simulink model "Joystick"  (R2017a)
settings: Solver=ode2  StartTime=0.0  StopTime=inf  FixedStep=0.001  RelTol=1e-3  EnableMultiTasking=on
model workspace (MAT data in the model file):
  Sig = Simulink.Signal
  Sig.DataType = 'auto'
  Sig.Dimensions = -1
  Sig.DimensionsMode = 'auto'
  Sig.Complexity = 'auto'
  Sig.SampleTime = -1
  Sig.SamplingMode = 'auto'
  video_step_size = 0.06
libraries: quarc_library x1
settings Model: SimulationMode=external  Creator=Admin  LastModifiedBy=mbohra
settings SolverCC: PositivePriorityOrder=on
settings OptimizationCC: LifeSpan=inf
settings DebuggingCC: ParameterPrecisionLossMsg=none  SFUnexpectedBacktrackingDiag=warning  SFNoUnconditionalDefaultTransitionDiag=warning  SFExecutionAtInitializationDiag=none
settings HardwareCC: ProdBitPerLong=64  ProdLargestAtomicFloat=None  ProdHWDeviceType=Intel->x86-64
settings RTWCC: SystemTargetFile=quarc_linux_x64.tlc  TemplateMakefile=quarc_linux_x64_tmf  Description=QUARC Linux x64 Target
settings STFCustomTargetCC: TargetLibSuffix=.a  TargetPreCompLibLocation=C:\PROGRA~3\QUARC\lib\2017a\LINUX_~1\release  ConcurrentExecutionCompliant=on  SystemTargetFile=quarc_linux_x64.tlc
settings GRTTargetCC: TargetLibSuffix=.a  TargetPreCompLibLocation=C:\PROGRA~3\QUARC\lib\2017a\LINUX_~1\release  TargetLangStandard=C89/C90 (ANSI)  ParMdlRefBuildCompliant=off  CompOptLevelCompliant=off  CombineOutputUpdateFcns=off  MatFileLogging=off  CPPClassGenCompliant=off  GRTInterface=on  UseToolchainInfoCompliant=off  ExtMode=on  ExtModeMexFile=quarc_comm  ExtModeMexArgs='-w -d /tmp -uri %u -IP_address tcpip://192.168.2.3:18666','tcpip://qondor888864.local:17002?retries=10'
settings ConfigComp: CovMetricSettings=dw  CovHtmlReporting=on  CovSaveCumulativeToWorkspaceVar=on  CovSaveSingleToWorkspaceVar=on  CovExternalEMLEnable=off

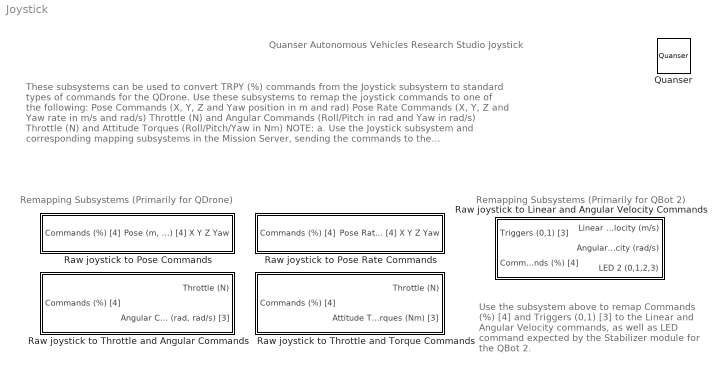
== system Joystick ==
  note: Remapping Subsystems (Primarily for QDrone)
  note: These subsystems can be used to convert TRPY (%) commands from the Joystick subsystem to standard types of commands for the QDrone. Use these subsystems to remap the joystick commands to one of the following:
      | Pose Commands (X, Y, Z and Yaw position in m and rad)
      | Pose Rate Commands (X, Y, Z and Yaw rate in m/s and rad/s)
      | Throttle (N) and Angular Commands (Roll/Pitch in rad and Yaw in rad/s)
      | Throttle (N) and Attitude Torques (Roll/Pitch/Yaw in Nm)
      |
      | NOTE:
      | a. Use the Joystick subsystem and corresponding mapping subsystems in the Mission Server, sending the commands to the Stabilizer/Commander on the QDrone with appropriate communication wrappers.
      | b. The Stabilizer module for the QDrone accepts command inputs for Throttle, Angular Commands and Attitude Torques.
      | c. The Commander module for the QDrone accepts command inputs for desired position.
  note: Quanser Autonomous Vehicles Research Studio
      | Joystick
  note: Remapping Subsystems (Primarily for QBot 2)
  note: Use the subsystem above to remap Commands (%) [4] and Triggers (0,1) [3] to the Linear and Angular Velocity commands, as well as LED command expected by the Stabilizer module for the QBot 2.
  Quanser : quarc_library/Logos/Quanser
  Raw joystick to Linear and Angular Velocity Commands : Subsystem
  Raw joystick to Pose Commands : Subsystem
  Raw joystick to Pose Rate Commands : Subsystem
  Raw joystick to Throttle and Angular Commands : Subsystem
  Raw joystick to Throttle and Torque Commands : Subsystem

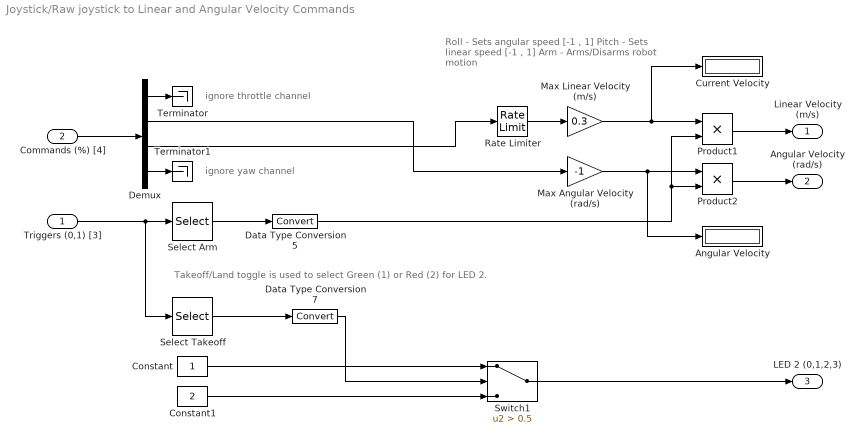
== system Joystick/Raw joystick to Linear and Angular Velocity Commands ==
  note: Takeoff/Land toggle is used to select Green (1) or Red (2) for LED 2.
  note: Roll		- Sets angular speed  	[-1		, 1]
      | Pitch	- Sets linear speed  	[-1		, 1]
      | Arm		- Arms/Disarms robot motion
  note: ignore throttle channel
  note: ignore yaw channel
  Triggers (0,1) [3] : Inport
  Commands (%) [4] : Inport  Port=2
  Angular Velocity : Display
  Constant : Constant
  Constant1 : Constant  Value=2
  Current Velocity : Display
  Data Type Conversion5 : DataTypeConversion
  Data Type Conversion7 : DataTypeConversion
  Demux : Demux
  Max Angular Velocity (rad/s) : Gain  Gain=-1
  Max Linear Velocity (m/s) : Gain  Gain=0.3
  Product1 : Product
  Product2 : Product
  Rate Limiter : RateLimiter  RisingSlewLimit=2  FallingSlewLimit=-2  SampleTimeMode=inherited
  Select Arm : Selector  InputPortWidth=3  IndexOptions=Index vector (dialog)  Indices=[1]  OutputSizes=1
  Select Takeoff : Selector  InputPortWidth=3  IndexOptions=Index vector (dialog)  Indices=[2]  OutputSizes=1
  Switch1 : Switch  Criteria=u2 > Threshold  Threshold=0.5
  Terminator : Terminator
  Terminator1 : Terminator
  Linear Velocity (m/s) : Outport  InitialOutput=0
  Angular Velocity (rad/s) : Outport  Port=2  InitialOutput=0
  LED 2 (0,1,2,3) : Outport  Port=3  InitialOutput=0
  wires:
  Commands (%) [4]/1 -> Demux/1
  Select Takeoff/1 -> Data Type Conversion7/1
  Switch1/1 -> LED 2 (0,1,2,3)/1
  Triggers (0,1) [3]/1 -> Select Takeoff/1, Select Arm/1
  Data Type Conversion7/1 -> Switch1/2
  Demux/4 -> Terminator1/1
  Data Type Conversion5/1 -> Product1/2, Product2/2
  Demux/3 -> Rate Limiter/1
  Demux/2 -> Max Angular Velocity (rad/s)/1
  Rate Limiter/1 -> Max Linear Velocity (m/s)/1
  Product2/1 -> Angular Velocity (rad/s)/1
  Constant1/1 -> Switch1/3
  Constant/1 -> Switch1/1
  Max Angular Velocity (rad/s)/1 -> Angular Velocity/1, Product2/1
  Product1/1 -> Linear Velocity (m/s)/1
  Demux/1 -> Terminator/1
  Max Linear Velocity (m/s)/1 -> Current Velocity/1, Product1/1
  Select Arm/1 -> Data Type Conversion5/1

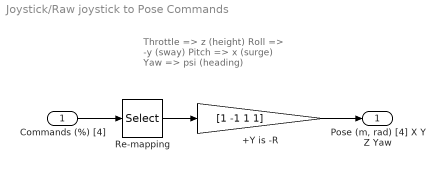
== system Joystick/Raw joystick to Pose Commands ==
  note: Throttle 	=> 	 z (height)
      | Roll 	=>	-y (sway)
      | Pitch	=> 	 x (surge)
      | Yaw		=> 	 psi (heading)
  Commands (%) [4] : Inport
  +Y is -R : Gain  Gain=[1 -1 1 1]
  Re-mapping : Selector  InputPortWidth=4  IndexOptions=Index vector (dialog)  Indices=[3 2 1 4]  OutputSizes=1
  "Pose (m, rad) [4] X Y Z Yaw" : Outport
  wires:
  +Y is -R/1 -> "Pose (m, rad) [4] X Y Z Yaw"/1
  Commands (%) [4]/1 -> Re-mapping/1
  Re-mapping/1 -> +Y is -R/1

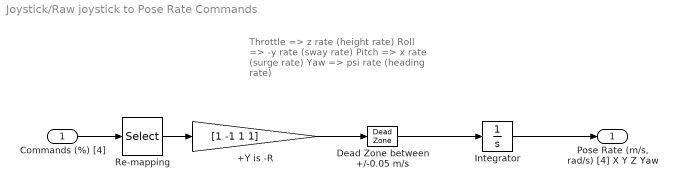
== system Joystick/Raw joystick to Pose Rate Commands ==
  note: Throttle 	=> 	 z rate (height rate)
      | Roll 	=>	-y rate (sway rate)
      | Pitch	=> 	 x rate (surge rate)
      | Yaw		=> 	 psi rate (heading rate)
  Commands (%) [4] : Inport
  +Y is -R : Gain  Gain=[1 -1 1 1]
  Dead Zone between +/-0.05 m/s : DeadZone  LowerValue=-0.05  UpperValue=0.05  SaturateOnIntegerOverflow=on
  Integrator : Integrator
  Re-mapping : Selector  InputPortWidth=4  IndexOptions=Index vector (dialog)  Indices=[3 2 1 4]  OutputSizes=1
  "Pose Rate (m/s, rad/s) [4] X Y Z Yaw" : Outport
  wires:
  Re-mapping/1 -> +Y is -R/1
  Commands (%) [4]/1 -> Re-mapping/1
  +Y is -R/1 -> Dead Zone between +/-0.05 m/s/1
  Integrator/1 -> "Pose Rate (m/s, rad/s) [4] X Y Z Yaw"/1
  Dead Zone between +/-0.05 m/s/1 -> Integrator/1

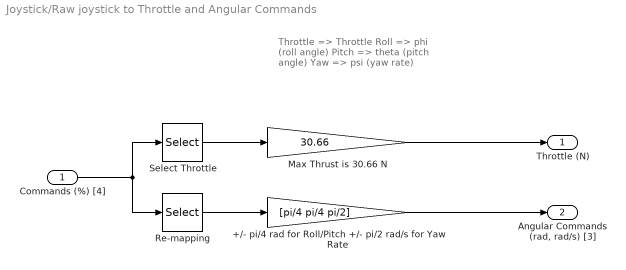
== system Joystick/Raw joystick to Throttle and Angular Commands ==
  note: Throttle 	=> 	 Throttle
      | Roll 	=>	 phi (roll angle)
      | Pitch	=> 	 theta (pitch angle)
      | Yaw		=> 	 psi (yaw rate)
  Commands (%) [4] : Inport
  +/- pi/4 rad for Roll/Pitch +/- pi/2 rad/s for Yaw Rate : Gain  Gain=[pi/4 pi/4 pi/2]
  Max Thrust is 30.66 N : Gain  Gain=30.66
  Re-mapping : Selector  InputPortWidth=4  IndexOptions=Index vector (dialog)  Indices=[2 3 4]  OutputSizes=1
  Select Throttle : Selector  InputPortWidth=4  IndexOptions=Index vector (dialog)  Indices=[1]  OutputSizes=1
  Throttle (N) : Outport
  "Angular Commands (rad, rad/s) [3]" : Outport  Port=2
  wires:
  +/- pi/4 rad for Roll/Pitch +/- pi/2 rad/s for Yaw Rate/1 -> "Angular Commands (rad, rad/s) [3]"/1
  Commands (%) [4]/1 -> Re-mapping/1, Select Throttle/1
  Re-mapping/1 -> +/- pi/4 rad for Roll/Pitch +/- pi/2 rad/s for Yaw Rate/1
  Select Throttle/1 -> Max Thrust is 30.66 N/1
  Max Thrust is 30.66 N/1 -> Throttle (N)/1

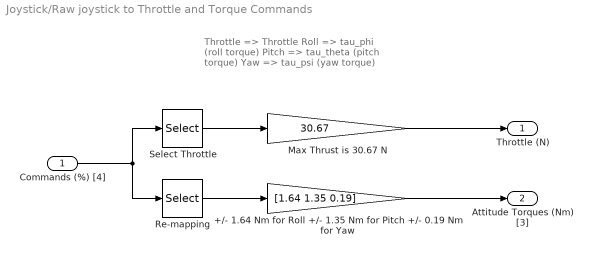
== system Joystick/Raw joystick to Throttle and Torque Commands ==
  note: Throttle 	=> 	 Throttle
      | Roll 	=>	 tau_phi (roll torque)
      | Pitch	=> 	 tau_theta (pitch torque)
      | Yaw		=> 	 tau_psi (yaw torque)
  Commands (%) [4] : Inport
  +/- 1.64 Nm for Roll +/- 1.35 Nm for Pitch +/- 0.19 Nm for Yaw : Gain  Gain=[1.64 1.35 0.19]
  Max Thrust is 30.67 N : Gain  Gain=30.67
  Re-mapping : Selector  InputPortWidth=4  IndexOptions=Index vector (dialog)  Indices=[2 3 4]  OutputSizes=1
  Select Throttle : Selector  InputPortWidth=4  IndexOptions=Index vector (dialog)  Indices=[1]  OutputSizes=1
  Throttle (N) : Outport
  Attitude Torques (Nm) [3] : Outport  Port=2
  wires:
  Max Thrust is 30.67 N/1 -> Throttle (N)/1
  Select Throttle/1 -> Max Thrust is 30.67 N/1
  Re-mapping/1 -> +/- 1.64 Nm for Roll +/- 1.35 Nm for Pitch +/- 0.19 Nm for Yaw/1
  Commands (%) [4]/1 -> Select Throttle/1, Re-mapping/1
  +/- 1.64 Nm for Roll +/- 1.35 Nm for Pitch +/- 0.19 Nm for Yaw/1 -> Attitude Torques (Nm) [3]/1
